simulink model "simple_roll"  (R2013a)
settings: Solver=ode45  StartTime=0.0  StopTime=10.0  RelTol=1e-3
values from neighbouring files (symbols this model uses):
  a = 2    [rocket_roll_validation.m]    (also in rocket_roll_validation_excess_code_not_pretty.m)
  b = 0.002    [rocket_roll_validation.m]    (also in rocket_roll_validation_excess_code_not_pretty.m; rotational_system.m; trail.m = 0.02)
  fr = 2.75*.0254    (= 0.06985)    [rocket_roll_validation.m]    (also in rocket_roll_validation_excess_code_not_pretty.m; rotational_system.m; trail.m)
  I = 0.0198    [rocket_roll_validation.m]    (also in rocket_roll_validation_excess_code_not_pretty.m; rotational_system.m; trail.m = 0.0197946818182)
  kp = .205    (= 0.205)    [rocket_roll_validation_excess_code_not_pretty.m]
  Tau = 0.02    [rocket_roll_validation.m]    (also in rocket_roll_validation_excess_code_not_pretty.m; rotational_system.m = 0.009)
libraries: simulink x1
settings Model: Creator=kenny  LastModifiedBy=kenny

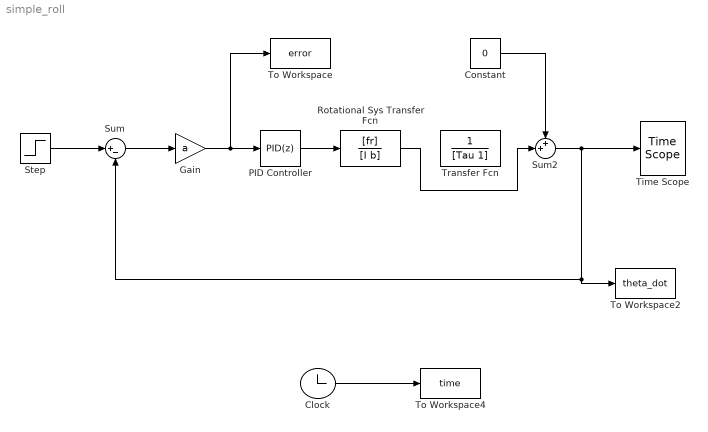
== system simple_roll ==
  Clock : Clock
  Constant : Constant  Value=0
  Gain : Gain  Gain=a
  PID Controller : simulink/Continuous/PID Controller  Controller=PID  TimeDomain=Discrete-time  SampleTime=.003  IntegratorMethod=Forward Euler  FilterMethod=Forward Euler  Form=Parallel  P=kp  I=0  D=0  N=100  InitialConditionSource=internal  InitialConditionForIntegrator=0  InitialConditionForFilter=0  ExternalReset=none  LimitOutput=off  UpperSaturationLimit=inf  LowerSaturationLimit=-inf  LinearizeAsGain=on  AntiWindupMode=none  Kb=1  TrackingMode=off  Kt=1  PParamMin=[]  PParamMax=[]  IParamMin=[]  IParamMax=[]  DParamMin=[]  DParamMax=[]  NParamMin=[]  NParamMax=[]  KbParamMin=[]  KbParamMax=[]  KtParamMin=[]  KtParamMax=[]  POutMin=[]  POutMax=[]  IOutMin=[]  IOutMax=[]  DOutMin=[]  DOutMax=[]  NOutMin=[]  NOutMax=[]  KbOutMin=[]  KbOutMax=[]  KtOutMin=[]  KtOutMax=[]  IntegratorOutMin=[]  IntegratorOutMax=[]  FilterOutMin=[]  FilterOutMax=[]  SumOutMin=[]  SumOutMax=[]  SumI1OutMin=[]  SumI1OutMax=[]  SumI2OutMin=[]  SumI2OutMax=[]  SumI3OutMin=[]  SumI3OutMax=[]  SumDOutMin=[]  SumDOutMax=[]  SaturationOutMin=[]  SaturationOutMax=[]  IntegratorContinuousStateAttributes=''  IntegratorStateMustResolveToSignalObject=off  IntegratorRTWStateStorageClass=Auto  FilterContinuousStateAttributes=''  FilterStateMustResolveToSignalObject=off  FilterRTWStateStorageClass=Auto
  Rotational Sys Transfer Fcn : TransferFcn  Numerator=[fr]  Denominator=[I b]
  Step : Step  Time=0  After=.51  SampleTime=0
  Sum : Sum  Inputs=|+-
  Sum2 : Sum  Inputs=++|
  Time Scope : TimeScope  DefaultConfigurationName=spbscopes.TimeScopeBlockCfg
      settings: CopyFcn=scopeextensions.ScopeBlock.callback(gcbh, 'onBlockCopy', gcbh);  DeleteFcn=scopeextensions.ScopeBlock.callback(gcbh, 'onBlockDelete');  PreSaveFcn=scopeextensions.ScopeBlock.callback(gcbh, 'onModelSave');  NameChangeFcn=scopeextensions.ScopeBlock.callback(gcbh, 'onBlockRename');  CloseFcn=scopeextensions.ScopeBlock.callback(gcbh, 'onBlockClose');  PreDeleteFcn=scopeextensions.ScopeBlock.callback(gcbh, 'onBlockPreDelete');
  To Workspace : ToWorkspace  VariableName=error  SampleTime=-1  SaveFormat=Structure With Time
  To Workspace2 : ToWorkspace  VariableName=theta_dot  SampleTime=-1  SaveFormat=Structure With Time
  To Workspace4 : ToWorkspace  VariableName=time  SampleTime=-1
  Transfer Fcn : TransferFcn  Denominator=[Tau 1]
  wires:
  Step/1 -> Sum/1
  Sum/1 -> Gain/1
  Gain/1 -> To Workspace/1, PID Controller/1
  Clock/1 -> To Workspace4/1
  Sum2/1 -> Sum/2, To Workspace2/1, Time Scope/1
  Constant/1 -> Sum2/1
  PID Controller/1 -> Rotational Sys Transfer Fcn/1
  Rotational Sys Transfer Fcn/1 -> Sum2/2
